simulink model "OuterLoop_Control"  (R2025a)
settings: configuration reference "csSingleInstance" (kept outside this file)
libraries: ControlLib x3, simulink x1
Description:
  | This model implements the outer loop controls (for pitch, roll, and yaw rate) of the helicopter flight control software.
settings Model: DataDictionary=DD_OuterLoop_Control.sldd  EnableAccessToBaseWorkspace=off  Creator=The MathWorks, Inc.  LastModifiedBy=The MathWorks, Inc.
settings ConfigSetRef: SourceName=csSingleInstance

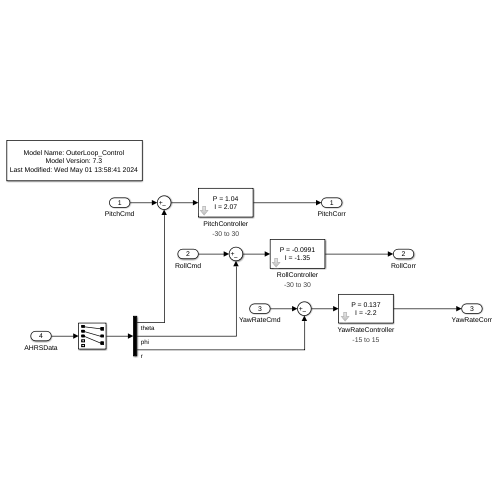
[thumbnail: Simulink's stored preview of the top-level diagram]
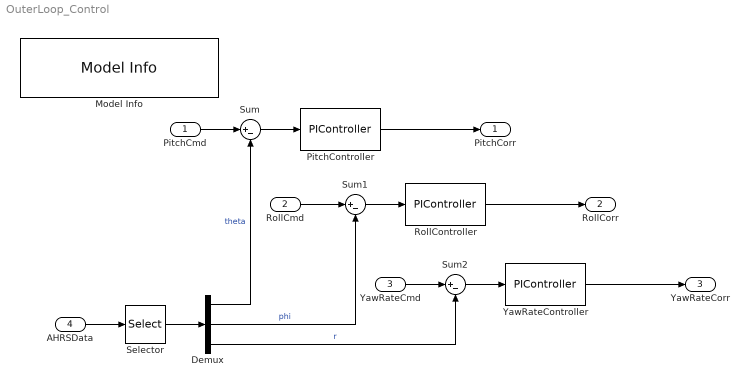
== system OuterLoop_Control ==
  PitchCmd : Inport  OutMin=-30  OutMax=30  OutDataTypeStr=double  PortDimensions=1  SampleTime=0.01
  RollCmd : Inport  Port=2  OutMin=-30  OutMax=30  OutDataTypeStr=double  PortDimensions=1  SampleTime=0.01
  YawRateCmd : Inport  Port=3  OutMin=-15  OutMax=15  OutDataTypeStr=double  PortDimensions=1  SampleTime=0.01
  AHRSData : Inport  Port=4  OutMin=-180  OutMax=180  OutDataTypeStr=double  PortDimensions=5  SampleTime=0.01
  Demux : Demux  Outputs=3
  Model Info : simulink/Model-Wide Utilities/Model Info  Frame=on  DisplayStringWithTags=|  HorizontalTextAlignment=Center  LeftAlignmentValue=0.5
      | Model Name: %<ModelName>
      | Model Version: %<ModelVersion>
      | Last Modified: %<LastModificationDate>
  PitchController : ControlLib/PIController  Tag=FilterWizardSubSystem  RequirementInfo={} %GIDa_f911a300_9a61_4411_9b01_11a22701fab0  kp=thetaKp  ki=thetaKi  hi=30  lo=-30  ts=0.01
      settings: AttributesFormatString=%<lo> to %<hi>
  RollController : ControlLib/PIController  Tag=FilterWizardSubSystem  RequirementInfo={} %GIDa_2f1be9ca_bc5b_4aa0_9327_ac3e34fc66a1  kp=phiKp  ki=phiKi  hi=30  lo=-30  ts=0.01
      settings: AttributesFormatString=%<lo> to %<hi>
  Selector : Selector  InputPortWidth=5  IndexOptions=Index vector (dialog)  Indices=[1 2 3]  OutputSizes=1
  Sum : Sum  Inputs=|+-  InputSameDT=on  OutDataTypeStr=Inherit: Same as first input
  Sum1 : Sum  Inputs=|+-  InputSameDT=on  OutDataTypeStr=Inherit: Same as first input
  Sum2 : Sum  Inputs=|+-  InputSameDT=on  OutDataTypeStr=Inherit: Same as first input
  YawRateController : ControlLib/PIController  Tag=FilterWizardSubSystem  RequirementInfo={} %GIDa_0dd42c5a_1833_4f1d_8e7b_15a3548c733a  kp=rKp  ki=rKi  hi=15  lo=-15  ts=0.01
      settings: AttributesFormatString=%<lo> to %<hi>
  PitchCorr : Outport  OutDataTypeStr=double  VectorParamsAs1DForOutWhenUnconnected=off
  RollCorr : Outport  Port=2  OutDataTypeStr=double  VectorParamsAs1DForOutWhenUnconnected=off
  YawRateCorr : Outport  Port=3  OutDataTypeStr=double  VectorParamsAs1DForOutWhenUnconnected=off
  wires:
  Selector/1 -> Demux/1
  Demux/1 -> Sum/2  "theta"
  Demux/2 -> Sum1/2  "phi"
  Demux/3 -> Sum2/2  "r"
  AHRSData/1 -> Selector/1
  PitchCmd/1 -> Sum/1
  RollCmd/1 -> Sum1/1
  YawRateCmd/1 -> Sum2/1
  Sum/1 -> PitchController/1
  PitchController/1 -> PitchCorr/1
  YawRateController/1 -> YawRateCorr/1
  Sum1/1 -> RollController/1
  RollController/1 -> RollCorr/1
  Sum2/1 -> YawRateController/1
